simulink model "platform_simulink_rejection_tracking"  (R2022a)
settings: Solver=VariableStepAuto  StartTime=0.0  StopTime=tfin  RelTol=1e-3
values from neighbouring files (symbols this model uses):
  Cy = [1 0 0 0]    [platform_disturbance_rejection.m]    (also in platform_disturbance_rejection_and_tracking.m; platform_simulink_rejection_and_tracking.m; platform_track_angle.m = [0 1 0 0]; platform_track_angle_with_integrator.m = [0 1 0 0])
  F = F_lmi(1:nx)    [platform_disturbance_rejection.m]    (also in platform_disturbance_rejection_and_tracking.m; platform_simulink_rejection_and_tracking.m; platform_track_angle.m = Ft(1,1:nx); platform_track_angle_with_integrator.m = Ftot(1,1:nx))
  Fq = F_lmi(nx+1:ny+nx)    [platform_disturbance_rejection.m]    (also in platform_disturbance_rejection_and_tracking.m; platform_simulink_rejection_and_tracking.m)
  parameters = [m,J,Ca,h,k]    [platform_disturbance_rejection.m]    (also in platform_disturbance_rejection_and_tracking.m; platform_regulation_finite_time_horizon.m; platform_regulation_infinite_time_horizon.m; platform_regulation_with_LMI.m)
  r = 0.1    [platform_disturbance_rejection_and_tracking.m]    (also in platform_simulink_rejection_and_tracking.m)
  Ts = 0.5    [platform_disturbance_rejection.m]    (also in platform_disturbance_rejection_and_tracking.m; platform_regulation_finite_time_horizon.m; platform_regulation_infinite_time_horizon.m; platform_regulation_with_LMI.m)
  ueq = op.Inputs.u    [platform_disturbance_rejection.m]    (also in platform_disturbance_rejection_and_tracking.m; platform_regulation_finite_time_horizon.m; platform_regulation_infinite_time_horizon.m; platform_regulation_with_LMI.m)
  x0 = [0;0;0;0]    [platform_disturbance_rejection.m]    (also in platform_disturbance_rejection_and_tracking.m; platform_regulation_finite_time_horizon.m; platform_regulation_infinite_time_horizon.m; platform_regulation_with_LMI.m)
  xeq = op.States.x    [platform_disturbance_rejection.m]    (also in platform_disturbance_rejection_and_tracking.m; platform_regulation_finite_time_horizon.m; platform_regulation_infinite_time_horizon.m; platform_regulation_with_LMI.m)
settings Model: Creator=User  LastModifiedBy=User

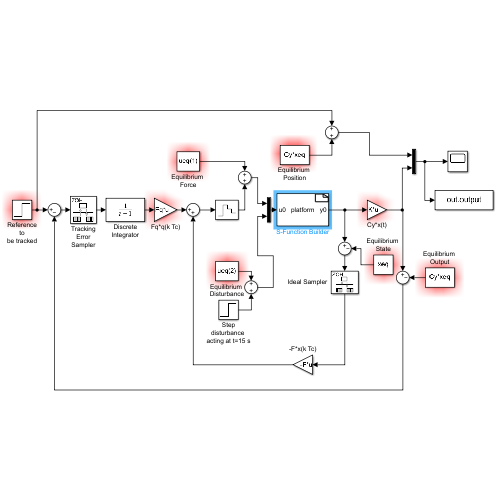
[thumbnail: Simulink's stored preview of the top-level diagram]
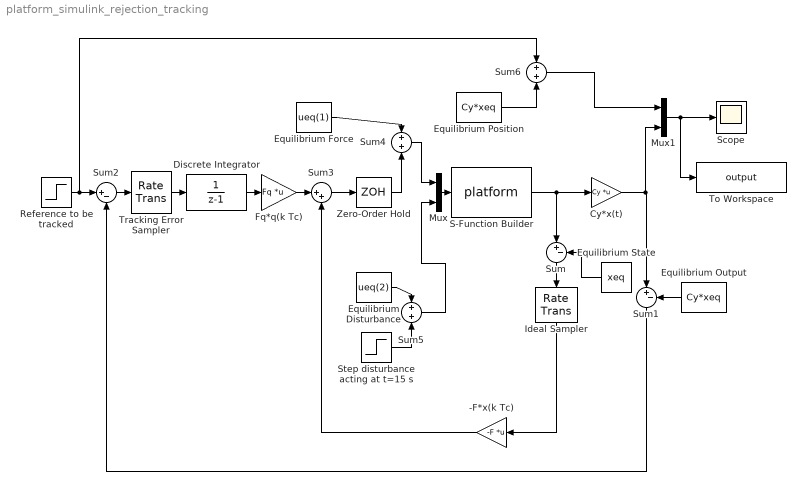
== system platform_simulink_rejection_tracking ==
  -F*x(k Tc) : Gain  Gain=-F  Multiplication=Matrix(K*u)
  Cy*x(t) : Gain  Gain=Cy  Multiplication=Matrix(K*u)
  Discrete Integrator : DiscreteTransferFcn  Denominator=[1 -1]  SampleTime=Ts
  Equilibrium Disturbance : Constant  Value=ueq(2)
  Equilibrium Force : Constant  Value=ueq(1)
  Equilibrium Output : Constant  Value=Cy*xeq
  Equilibrium Position : Constant  Value=Cy*xeq
  Equilibrium State : Constant  Value=xeq
  Fq*q(k Tc) : Gain  Gain=Fq  Multiplication=Matrix(K*u)
  Ideal Sampler : RateTransition  OutPortSampleTime=Ts
  Mux : Mux  Inputs=2
  Mux1 : Mux  Inputs=2
  Reference to be tracked : Step  Time=0  After=r  SampleTime=0
  S-Function Builder : S-Function  FunctionName=platform  Parameters=x0,parameters  SFunctionModules=platform_wrapper  SFunctionDeploymentMode=off  EnableBusSupport=off  mask(S-Function Builder){}
      mask help: Simulink:masks:SFunctionBuilder_MD
      mask init:
      | val = [[.9  0.75 0.75 1 1 .9 .9 1]',[1 1 0.75 0.75 .9 .9 1 .9]'];try , sys = get_param(gcb,'SfunBuilderFcnName');if isempty(sys), sys = get_param(gcb,'FunctionName'); end,catch, sys = get_param(gcb,'FunctionName'); end
      settings: CopyFcn=set_param(gcbh,'LinkStatus','none')  OpenFcn=sfunctionwizard(gcbh)
      mask Display: plot(val(:,1),val(:,2)),disp(sys),port_label('input',1,'u0'),port_label('output',1,'y0')
  Scope : Scope
  Step disturbance acting at t=15 s : Step  Time=15  SampleTime=0
  Sum : Sum  Inputs=|+-
  Sum1 : Sum  Inputs=|+-
  Sum2 : Sum  Inputs=|+-
  Sum3 : Sum  Inputs=|++
  Sum4 : Sum
  Sum5 : Sum
  Sum6 : Sum
  To Workspace : ToWorkspace  VariableName=output  SampleTime=-1
  Tracking Error Sampler : RateTransition  OutPortSampleTime=Ts
  Zero-Order Hold : ZeroOrderHold  SampleTime=-1
  wires:
  Reference to be tracked/1 -> Sum6/1, Sum2/1
  Sum2/1 -> Tracking Error Sampler/1
  Tracking Error Sampler/1 -> Discrete Integrator/1
  Mux/1 -> S-Function Builder/1
  Sum5/1 -> Mux/2
  Sum4/1 -> Mux/1
  Discrete Integrator/1 -> Fq*q(k Tc)/1
  Fq*q(k Tc)/1 -> Sum3/1
  Sum3/1 -> Zero-Order Hold/1
  Equilibrium Force/1 -> Sum4/1
  Zero-Order Hold/1 -> Sum4/2
  Equilibrium Disturbance/1 -> Sum5/1
  Step disturbance acting at t=15 s/1 -> Sum5/2
  Sum/1 -> Ideal Sampler/1
  S-Function Builder/1 -> Sum/1, Cy*x(t)/1
  Equilibrium State/1 -> Sum/2
  -F*x(k Tc)/1 -> Sum3/2
  Ideal Sampler/1 -> -F*x(k Tc)/1
  Equilibrium Output/1 -> Sum1/2
  Mux1/1 -> To Workspace/1, Scope/1
  Cy*x(t)/1 -> Sum1/1, Mux1/2
  Equilibrium Position/1 -> Sum6/2
  Sum6/1 -> Mux1/1
  Sum1/1 -> Sum2/2
